simulink library "DaidalusV201Block"  (R2018b)
settings: Solver=VariableStepAuto  StartTime=0.0  StopTime=10.0  RelTol=1e-3
undefined symbols (not defined in the file or in its folder): daa_caFactor, daa_corrDTHR, daa_corrEarly, daa_corrLookahead, daa_corrTCOA, daa_corrTTHR, daa_corrZTHR, daa_guideDTHR, daa_guideLookahead, daa_guideTCOA, daa_guideTTHR, daa_guideZTHR, daa_minAlt, daa_minHorRec, daa_prevDTHR, daa_prevEarly, daa_prevLookahead, daa_prevTCOA, daa_prevTTHR, daa_prevZTHR, daa_recStabTime, daa_singleDirRecovery, daa_warnDTHR, daa_warnEarly, daa_warnLookahead, daa_warnTCOA, daa_warnTTHR, daa_warnZTHR, DEGAS
settings Model: Creator=RA24876  LastModifiedBy=PE29732
settings SFSimCC: SimUseLocalCustomCode=off
settings RTWCC: RTWUseLocalCustomCode=off
settings CodeAppCC: StateflowObjectComments=on

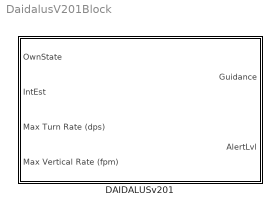
== system DaidalusV201Block ==
  DAIDALUSv201 : Subsystem  mask(DAIDALUS){DTHR=daa_guideDTHR, ZTHR=daa_guideZTHR, TTHR=daa_guideTTHR, TCOA=daa_guideTCOA, lookahead_time=daa_guideLookahead, use_single_direction=daa_singleDirRecovery, prev_DTHR=daa_prevDTHR, prev_ZTHR=daa_prevZTHR, prev_TTHR=daa_prevTTHR, prev_TCOA=daa_prevTCOA, prev_lookahead=daa_prevLookahead, prev_early=daa_prevEarly, corr_DTHR=daa_corrDTHR, corr_ZTHR=daa_corrZTHR, corr_TTHR=daa_corrTTHR, corr_TCOA=daa_corrTCOA, corr_lookahead=daa_corrLookahead, corr_early=daa_corrEarly, warn_DTHR=daa_warnDTHR, warn_ZTHR=daa_warnZTHR, warn_TTHR=daa_warnTTHR, warn_TCOA=daa_warnTCOA, warn_lookahead=daa_warnLookahead, warn_early=daa_warnEarly, min_alt=daa_minAlt, rec_stab_time=daa_recStabTime, min_hor_rec=daa_minHorRec, ca_factor=daa_caFactor}
      mask prompts: DTHR "DTHR (ft)"; ZTHR "ZTHR (ft)"; TTHR "TTHR (s)"; TCOA "TCOA (s)"; lookahead_time "Guidance Lookahead Time"; use_single_direction "Use Single Direction for Recovery Guidance?"; prev_DTHR "DTHR (ft)"; prev_ZTHR "ZTHR (ft)"; prev_TTHR "TTHR (s)"; prev_TCOA "TCOA (s)"; prev_lookahead "Lookahead Time (s)"; prev_early "Early Threshold (s)"; corr_DTHR "DTHR (ft)"; corr_ZTHR "ZTHR (ft)"; corr_TTHR "TTHR (s)"; corr_TCOA "TCOA (s)"; corr_lookahead "Lookahead Time (s)"; corr_early "Early Threshold (s)"; warn_DTHR "DTHR (ft)"; warn_ZTHR "ZTHR (ft)"; warn_TTHR "TTHR (s)"; warn_TCOA "TCOA (s)"; warn_lookahead "Lookahead Time (s)"; warn_early "Early Threshold (s)"; min_alt "Minimum Altitude (ft)"; rec_stab_time "Recovery Stability Time (s)"; min_hor_rec "Min. Horizontal Recovery Distance (ft)"; ca_factor "Collision Avoidance Factor"
      mask help:
      | S-function interface with DAIDALUS v1.a0 for DAA alerting and suggestive guidance.  Parameters may be set with wrapper class Daidalus.
      |
      | Input signals are the ownship state (AircraftState bus), the intruder state (AircraftEstimate bus), and maximum ownship turn rate and vertical rate.  Output signals are the alert level (0-3) and guidance as a 283-element array.
      mask Help:
      | S-function interface with DAIDALUS for DAA alerting and suggestive guidance.  Parameters may be set with wrapper class Daidalus.
      | 
      | Input signals are the ownship state (AircraftState bus), the intruder state (AircraftEstimate bus), and maximum ownship turn rate and vertical rate.
      | Output signals are the alert level (0-3) and guidance as a 283-element array.  The first 271 elements contain track guidance for headings -135 deg to 135 deg from the ownship's current heading.  The remaining elements are altitude/guidance pairs.  Guidance values are 0 for conflict-free, 1 for well clear recovery, and 2-4 for conflict.
      | 
      | Randal Guendel, 21 September 2016
      mask DialogControl Container4 Prompt: Guidance
      mask DialogControl Control3 Prompt: Conflict Region Definition:
      mask DialogControl Container5 Prompt: Alerting
      mask DialogControl Control2 Prompt: Preventive Alert Definition:
      mask DialogControl Control4 Prompt: Corrective Alert Definition:
      mask DialogControl Control5 Prompt: Warning Alert Definition:
      mask DialogControl Container6 Prompt: Bands Parameters
      mask DialogControl Control7 Prompt: Conflict Bands Parameters:
      mask DialogControl Control8 Prompt: Recovery Bands Parameters:

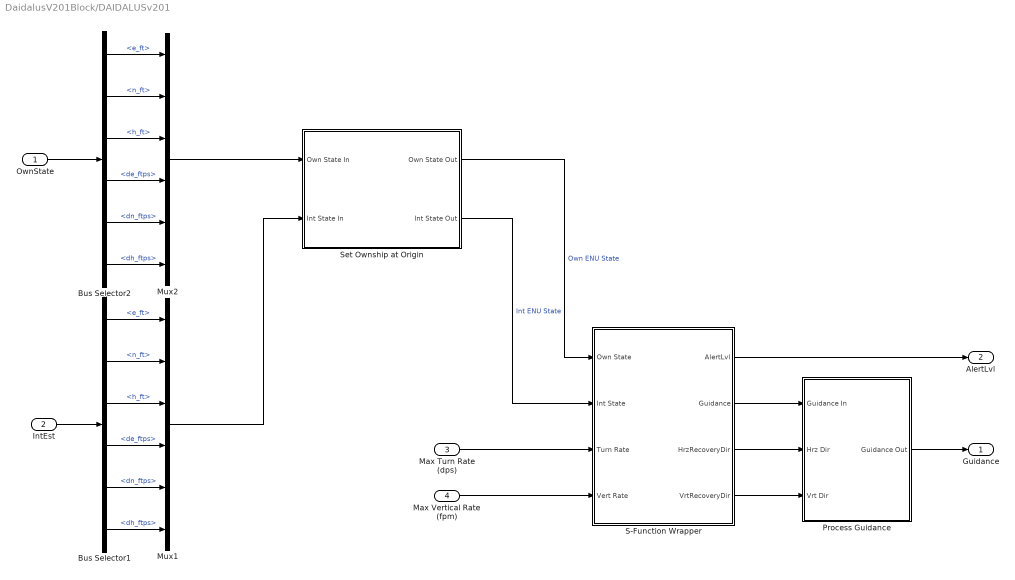
== system DaidalusV201Block/DAIDALUSv201 ==
  OwnState : Inport  OutDataTypeStr=Bus: AircraftEstimate
  IntEst : Inport  Port=2  OutDataTypeStr=Bus: AircraftEstimate
  Max Turn Rate (dps) : Inport  Port=3
  Max Vertical Rate (fpm) : Inport  Port=4
  Bus Selector1 : BusSelector  OutputSignals=enuStateEstimate.e_ft,enuStateEstimate.n_ft,enuStateEstimate.h_ft,enuStateEstimate.de_ftps,enuStateEstimate.dn_ftps,enuStateEstimate.dh_ftps
  Bus Selector2 : BusSelector  OutputSignals=enuStateEstimate.e_ft,enuStateEstimate.n_ft,enuStateEstimate.h_ft,enuStateEstimate.de_ftps,enuStateEstimate.dn_ftps,enuStateEstimate.dh_ftps
  Mux1 : Mux  Inputs=6
  Mux2 : Mux  Inputs=6
  Process Guidance : Subsystem
  S-Function Wrapper : Subsystem
  Set Ownship at Origin : Subsystem
  Guidance : Outport
  AlertLvl : Outport  Port=2
  wires:
  Process Guidance/1(Guidance Out) -> Guidance/1
  S-Function Wrapper/4(VrtRecoveryDir) -> Process Guidance/3(Vrt Dir)
  S-Function Wrapper/3(HrzRecoveryDir) -> Process Guidance/2(Hrz Dir)
  S-Function Wrapper/2(Guidance) -> Process Guidance/1(Guidance In)
  S-Function Wrapper/1(AlertLvl) -> AlertLvl/1
  Max Vertical Rate (fpm)/1 -> S-Function Wrapper/4(Vert Rate)
  Max Turn Rate (dps)/1 -> S-Function Wrapper/3(Turn Rate)
  Set Ownship at Origin/2(Int State Out) -> S-Function Wrapper/2(Int State)  "Int ENU State"
  Set Ownship at Origin/1(Own State Out) -> S-Function Wrapper/1(Own State)  "Own ENU State"
  OwnState/1 -> Bus Selector2/1
  Bus Selector1/6 -> Mux1/6  "<dh_ftps>"
  Bus Selector1/3 -> Mux1/3  "<h_ft>"
  IntEst/1 -> Bus Selector1/1
  Mux1/1 -> Set Ownship at Origin/2(Int State In)
  Bus Selector1/1 -> Mux1/1  "<e_ft>"
  Bus Selector1/2 -> Mux1/2  "<n_ft>"
  Bus Selector1/4 -> Mux1/4  "<de_ftps>"
  Bus Selector1/5 -> Mux1/5  "<dn_ftps>"
  Bus Selector2/1 -> Mux2/1  "<e_ft>"
  Bus Selector2/2 -> Mux2/2  "<n_ft>"
  Bus Selector2/3 -> Mux2/3  "<h_ft>"
  Bus Selector2/4 -> Mux2/4  "<de_ftps>"
  Bus Selector2/5 -> Mux2/5  "<dn_ftps>"
  Bus Selector2/6 -> Mux2/6  "<dh_ftps>"
  Mux2/1 -> Set Ownship at Origin/1(Own State In)

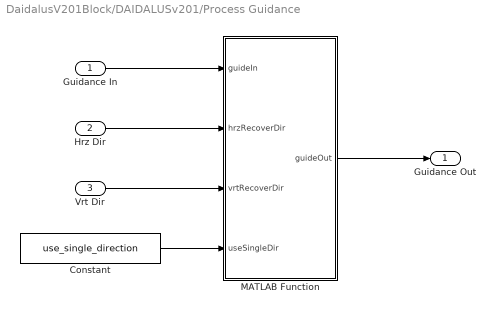
== system DaidalusV201Block/DAIDALUSv201/Process Guidance ==
  Guidance In : Inport
  Hrz Dir : Inport  Port=2
  Vrt Dir : Inport  Port=3
  Constant : Constant  Value=use_single_direction
  MATLAB Function : MATLAB Function  TreatAsAtomicUnit=on
  Guidance Out : Outport
  wires:
  Constant/1 -> MATLAB Function/4(useSingleDir)
  Vrt Dir/1 -> MATLAB Function/3(vrtRecoverDir)
  Hrz Dir/1 -> MATLAB Function/2(hrzRecoverDir)
  MATLAB Function/1(guideOut) -> Guidance Out/1
  Guidance In/1 -> MATLAB Function/1(guideIn)

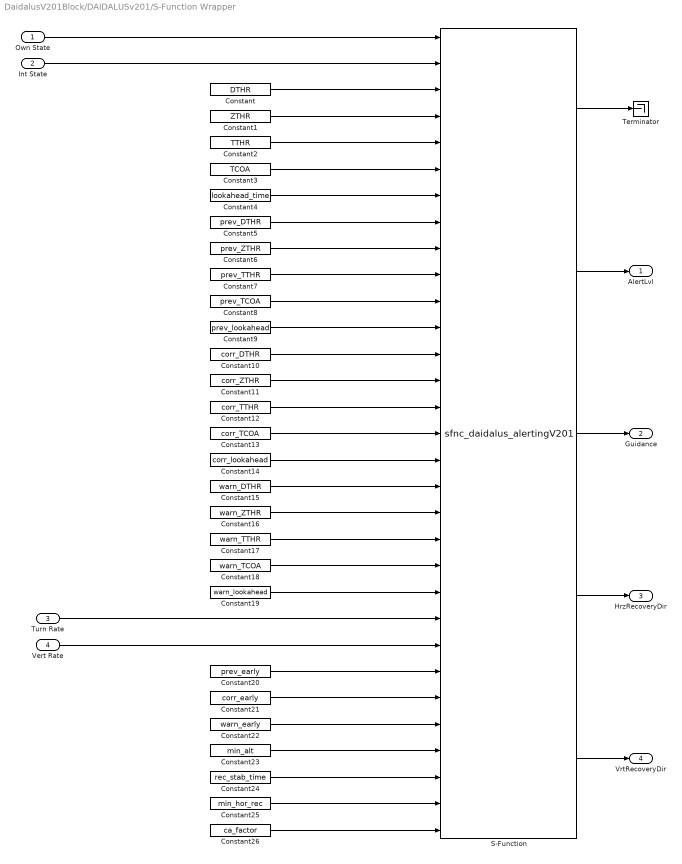
== system DaidalusV201Block/DAIDALUSv201/S-Function Wrapper ==
  Own State : Inport
  Int State : Inport  Port=2
  Turn Rate : Inport  Port=3
  Vert Rate : Inport  Port=4
  Constant : Constant  Value=DTHR
  Constant1 : Constant  Value=ZTHR
  Constant10 : Constant  Value=corr_DTHR
  Constant11 : Constant  Value=corr_ZTHR
  Constant12 : Constant  Value=corr_TTHR
  Constant13 : Constant  Value=corr_TCOA
  Constant14 : Constant  Value=corr_lookahead
  Constant15 : Constant  Value=warn_DTHR
  Constant16 : Constant  Value=warn_ZTHR
  Constant17 : Constant  Value=warn_TTHR
  Constant18 : Constant  Value=warn_TCOA
  Constant19 : Constant  Value=warn_lookahead
  Constant2 : Constant  Value=TTHR
  Constant20 : Constant  Value=prev_early
  Constant21 : Constant  Value=corr_early
  Constant22 : Constant  Value=warn_early
  Constant23 : Constant  Value=min_alt
  Constant24 : Constant  Value=rec_stab_time
  Constant25 : Constant  Value=min_hor_rec
  Constant26 : Constant  Value=ca_factor
  Constant3 : Constant  Value=TCOA
  Constant4 : Constant  Value=lookahead_time
  Constant5 : Constant  Value=prev_DTHR
  Constant6 : Constant  Value=prev_ZTHR
  Constant7 : Constant  Value=prev_TTHR
  Constant8 : Constant  Value=prev_TCOA
  Constant9 : Constant  Value=prev_lookahead
  S-Function : S-Function  FunctionName=sfnc_daidalus_alertingV201  SFunctionModules=sfnc_daidalus_alertingV201 DaidalusAlertAndGuidance  SFunctionDeploymentMode=off  EnableBusSupport=off
  Terminator : Terminator
  AlertLvl : Outport
  Guidance : Outport  Port=2
  HrzRecoveryDir : Outport  Port=3
  VrtRecoveryDir : Outport  Port=4
  wires:
  Constant26/1 -> S-Function/31
  Constant25/1 -> S-Function/30
  Constant24/1 -> S-Function/29
  Constant23/1 -> S-Function/28
  Constant22/1 -> S-Function/27
  Constant21/1 -> S-Function/26
  Constant20/1 -> S-Function/25
  S-Function/4 -> HrzRecoveryDir/1
  Own State/1 -> S-Function/1
  Int State/1 -> S-Function/2
  S-Function/3 -> Guidance/1
  S-Function/2 -> AlertLvl/1
  Constant13/1 -> S-Function/16
  Constant12/1 -> S-Function/15
  Constant11/1 -> S-Function/14
  Constant10/1 -> S-Function/13
  Constant9/1 -> S-Function/12
  Constant8/1 -> S-Function/11
  Constant1/1 -> S-Function/4
  Constant2/1 -> S-Function/5
  Constant3/1 -> S-Function/6
  Constant7/1 -> S-Function/10
  Constant6/1 -> S-Function/9
  Constant5/1 -> S-Function/8
  Constant4/1 -> S-Function/7
  Constant/1 -> S-Function/3
  S-Function/1 -> Terminator/1
  Constant14/1 -> S-Function/17
  Constant15/1 -> S-Function/18
  Vert Rate/1 -> S-Function/24
  Constant19/1 -> S-Function/22
  Turn Rate/1 -> S-Function/23
  Constant18/1 -> S-Function/21
  Constant17/1 -> S-Function/20
  Constant16/1 -> S-Function/19
  S-Function/5 -> VrtRecoveryDir/1

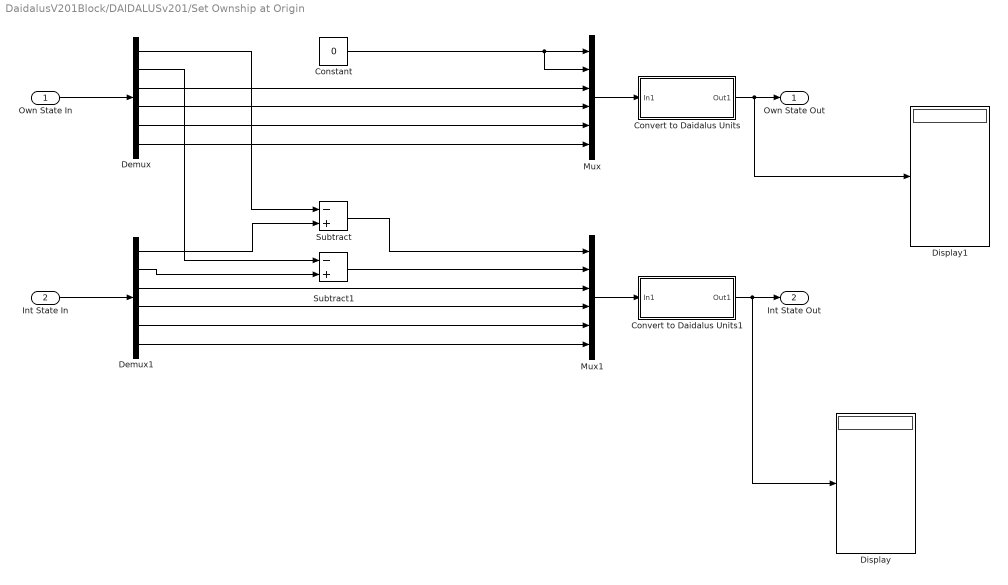
== system DaidalusV201Block/DAIDALUSv201/Set Ownship at Origin ==
  Own State In : Inport
  Int State In : Inport  Port=2
  Constant : Constant  Value=0
  Convert to Daidalus Units : Subsystem
  Convert to Daidalus Units1 : Subsystem
  Demux : Demux  Outputs=6
  Demux1 : Demux  Outputs=6
  Display : Display
  Display1 : Display
  Mux : Mux  Inputs=6
  Mux1 : Mux  Inputs=6
  Subtract : Sum  Inputs=-+
  Subtract1 : Sum  Inputs=-+
  Own State Out : Outport
  Int State Out : Outport  Port=2
  wires:
  Demux1/1 -> Subtract/2
  Demux1/2 -> Subtract1/2
  Subtract1/1 -> Mux1/2
  Subtract/1 -> Mux1/1
  Demux1/3 -> Mux1/3
  Demux1/4 -> Mux1/4
  Demux1/5 -> Mux1/5
  Demux1/6 -> Mux1/6
  Demux/2 -> Subtract1/1
  Demux/1 -> Subtract/1
  Constant/1 -> Mux/1, Mux/2
  Demux/3 -> Mux/3
  Demux/4 -> Mux/4
  Demux/5 -> Mux/5
  Demux/6 -> Mux/6
  Mux1/1 -> Convert to Daidalus Units1/1(In1)
  Mux/1 -> Convert to Daidalus Units/1(In1)
  Int State In/1 -> Demux1/1
  Own State In/1 -> Demux/1
  Convert to Daidalus Units/1(Out1) -> Display1/1, Own State Out/1
  Convert to Daidalus Units1/1(Out1) -> Display/1, Int State Out/1

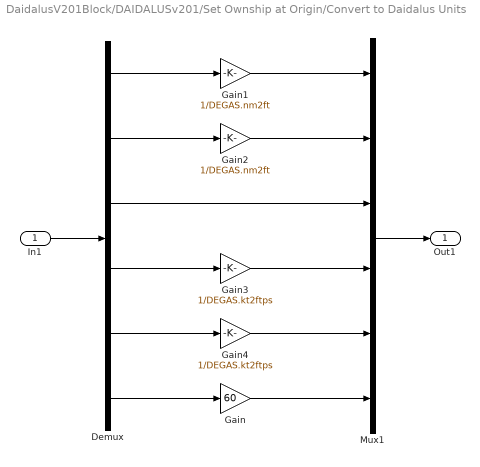
== system DaidalusV201Block/DAIDALUSv201/Set Ownship at Origin/Convert to Daidalus Units ==
  In1 : Inport
  Demux : Demux  Outputs=6
  Gain : Gain  Gain=60
  Gain1 : Gain  Gain=1/DEGAS.nm2ft
  Gain2 : Gain  Gain=1/DEGAS.nm2ft
  Gain3 : Gain  Gain=1/DEGAS.kt2ftps
  Gain4 : Gain  Gain=1/DEGAS.kt2ftps
  Mux1 : Mux  Inputs=6
  Out1 : Outport
  wires:
  Mux1/1 -> Out1/1
  Demux/6 -> Gain/1
  Demux/1 -> Gain1/1
  Demux/2 -> Gain2/1
  Demux/3 -> Mux1/3
  Demux/4 -> Gain3/1
  Demux/5 -> Gain4/1
  In1/1 -> Demux/1
  Gain/1 -> Mux1/6
  Gain1/1 -> Mux1/1
  Gain2/1 -> Mux1/2
  Gain3/1 -> Mux1/4
  Gain4/1 -> Mux1/5

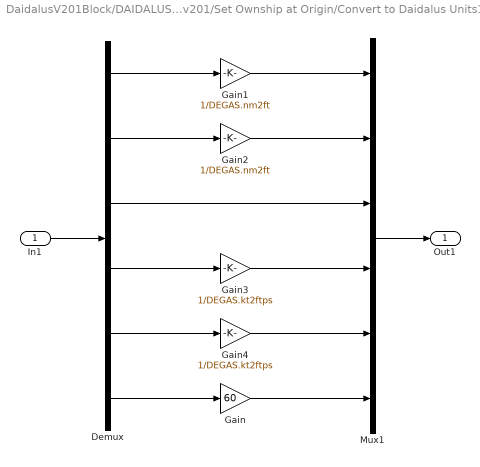
== system DaidalusV201Block/DAIDALUSv201/Set Ownship at Origin/Convert to Daidalus Units1 ==
  In1 : Inport
  Demux : Demux  Outputs=6
  Gain : Gain  Gain=60
  Gain1 : Gain  Gain=1/DEGAS.nm2ft
  Gain2 : Gain  Gain=1/DEGAS.nm2ft
  Gain3 : Gain  Gain=1/DEGAS.kt2ftps
  Gain4 : Gain  Gain=1/DEGAS.kt2ftps
  Mux1 : Mux  Inputs=6
  Out1 : Outport
  wires:
  Mux1/1 -> Out1/1
  Demux/6 -> Gain/1
  Demux/1 -> Gain1/1
  Demux/2 -> Gain2/1
  Demux/3 -> Mux1/3
  Demux/4 -> Gain3/1
  Demux/5 -> Gain4/1
  In1/1 -> Demux/1
  Gain/1 -> Mux1/6
  Gain1/1 -> Mux1/1
  Gain2/1 -> Mux1/2
  Gain3/1 -> Mux1/4
  Gain4/1 -> Mux1/5

== matlab function DaidalusV201Block/DAIDALUSv201/Process Guidance/MATLAB Function ==
  data: guideIn input; guideOut output; hrzRecoverDir input; vrtRecoverDir input; useSingleDir input
function guideOut = fcn(guideIn, hrzRecoverDir, vrtRecoverDir, useSingleDir)
%#codegen

guideOut = DaidalusV201_ExternalFunctions.processGuidance(guideIn, hrzRecoverDir, vrtRecoverDir, useSingleDir);
